simulink model "p221"  (R2018b)
settings: Solver=VariableStepAuto  StartTime=0.0  StopTime=40.0  RelTol=1e-3
settings Model: Creator=mikiz  LastModifiedBy=mikiz

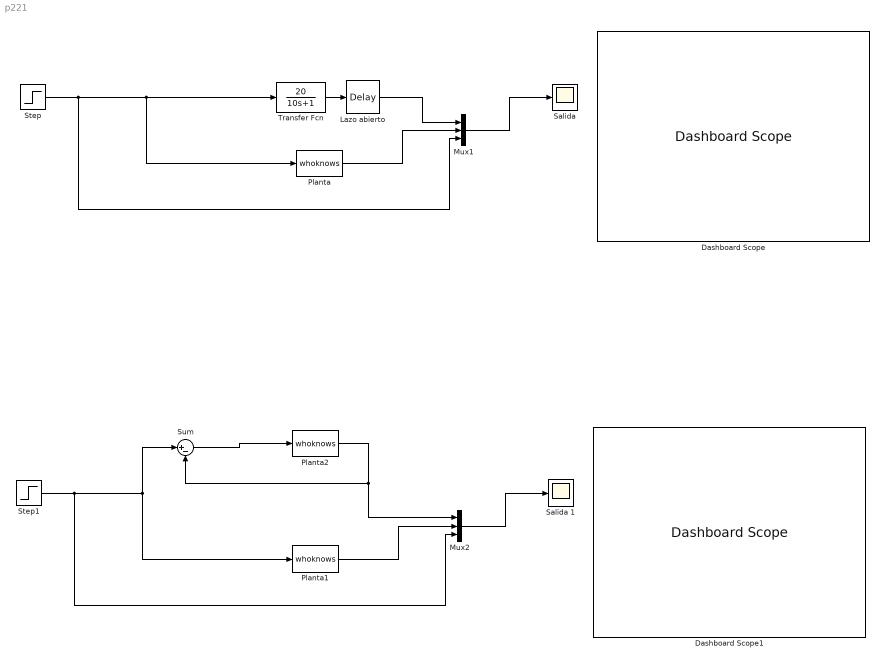
== system p221 ==
  Dashboard Scope : DashboardScope  WebBlockId=1
  Dashboard Scope1 : DashboardScope  WebBlockId=8
  Lazo abierto : TransportDelay  DelayTime=2
  Mux1 : Mux  Inputs=3
  Mux2 : Mux  Inputs=3
  Planta : M-S-Function  FunctionName=whoknows  Parameters=L, P1, P2, T, R  mask{L=7, P1=0, P2=7, T=1, R=0}
      mask prompts: L "Laboratorio"; P1 "Primer digito del Puesto"; P2 "Segundo digito del Puesto"; T "Tipo de Planta"; R "Ruido"
      mask Display: disp('Sistema')
  Planta1 : M-S-Function  FunctionName=whoknows  Parameters=L, P1, P2, T, R  mask{L=7, P1=0, P2=7, T=1, R=0}
      mask prompts: L "Laboratorio"; P1 "Primer digito del Puesto"; P2 "Segundo digito del Puesto"; T "Tipo de Planta"; R "Ruido"
      mask Display: disp('Sistema')
  Planta2 : M-S-Function  FunctionName=whoknows  Parameters=L, P1, P2, T, R  mask{L=7, P1=0, P2=7, T=2, R=0}
      mask prompts: L "Laboratorio"; P1 "Primer digito del Puesto"; P2 "Segundo digito del Puesto"; T "Tipo de Planta"; R "Ruido"
      mask Display: disp('Sistema')
  "Salida " : Scope
  Salida 1 : Scope
  Step : Step  SampleTime=0
  Step1 : Step  SampleTime=0
  Sum : Sum  Inputs=|+-
  Transfer Fcn : TransferFcn  Numerator=[20]  Denominator=[10 1]
  wires:
  Step/1 -> Mux1/3, Planta/1, Transfer Fcn/1
  Transfer Fcn/1 -> Lazo abierto/1
  Lazo abierto/1 -> Mux1/1
  Mux1/1 -> "Salida "/1
  Planta/1 -> Mux1/2
  Planta1/1 -> Mux2/2
  Step1/1 -> Mux2/3, Planta1/1, Sum/1
  Mux2/1 -> Salida 1/1
  Sum/1 -> Planta2/1
  Planta2/1 -> Sum/2, Mux2/1
